simulink model "ADIA"  (R2018b)
settings: Solver=FixedStepDiscrete  StartTime=0.0  StopTime=10.0  FixedStep=0.02  RelTol=1e-3
undefined symbols (not defined in the file or in its folder): ACC_State_Active, ACC_State_BrakeOnly, ACC_State_Suspended, ACC_State_WaitingRise, ADAS_AEBBrakingProg, ADAS_DeclControlReq, ADAS_DriveOff, ADAS_ESCHoldReq_NotHold, ADASDecType_ACC, ADASDecType_AEB, ADIA_ACC_Acceleration_OOR_DecCount_C, ADIA_ACC_Acceleration_OOR_Duration_C, ADIA_ACC_Acceleration_OOR_IncCount_C, ADIA_ACC_Acceleration_OOR_LLim_C, ADIA_ACC_Acceleration_OOR_ULim_C, ADIA_ACC_AccelTrqReq_MixedDia_ULim_C, ADIA_ACC_AccelTrqReq_ULim_C, ADIA_ACC_Deceleration_Mixed_ULim_C, ADIA_ACC_Deceleration_OOR_DecCount_C, ADIA_ACC_Deceleration_OOR_Duration_C, ADIA_ACC_Deceleration_OOR_IncCount_C, ADIA_ACC_Deceleration_OOR_LLim_C, ADIA_ACC_Deceleration_OOR_ULim_C, ADIA_ACC_DriveOff_Distance_C, ADIA_ACC_DriveOff_TimeLim_C, ADIA_ACC_ReqMixed_DecCount_C, ADIA_ACC_ReqMixed_Duration_C, ADIA_ACC_ReqMixed_IncCount_C, ADIA_AccPedalRaw_MaxLim_C, ADIA_AccPedalRaw_MinLim_C, ADIA_ADAS_HoldDecReq_Set_C, ADIA_ADAS_HoldRConfirm_TimeLim_C, ADIA_ADAS_HoldVehSpd_Lim_C, ADIA_AEB_VehSpdDec_LLim_C, ADIA_AEB_VehSpdDec_ULim_C, ADIA_ASWFault_OvrdEn_C, ADIA_ASWFault_OvrdValue_C, ADIA_BatteryOutOfRange_DecCount_C, ADIA_BatteryOutOfRange_Duration_C, ADIA_BatteryOutOfRange_IncCount_C, ADIA_BattVolt_MaxLim_C, ADIA_BattVolt_MinLim_C, ADIA_BCM3_33C_InvBrkLight_DecCount_C, ADIA_BCM3_33C_InvBrkLight_Duration_C, ADIA_BCM3_33C_InvBrkLight_IncCount_C, ADIA_BCM_BattVolt_OvrdEn_C, ADIA_BCM_BattVolt_OvrdVal_C, ADIA_BCM_BrakeLampStaus_OvrdEn_C, ADIA_BCM_BrakeLampStaus_OvrdVal_C, ADIA_BCM_CHMSLStaus_OvrdEn_C, ADIA_BCM_CHMSLStaus_OvrdVal_C, ADIA_BCM_LeftTurnSwSt_OvrdEn_C, ADIA_BCM_LeftTurnSwSt_OvrdVal_C, ADIA_BCM_RightTurnSwSt_OvrdEn_C, ADIA_BCM_RightTurnSwSt_OvrdVal_C, ADIA_BCM_TurnSwFailure_DecCount_C, ADIA_BCM_TurnSwFailure_Duration_C, ADIA_BCM_TurnSwFailure_IncCount_C, ADIA_BSWFault_Ignore_C, ADIA_BSWFault_OvrdEn_C ... (+281)
libraries: simulink x208
(part 5 of 10)

== system ADIA/ADAS_Diagnostics/Diagnostics_Processing/DTC_ACC_HoldConfirm_Safety_Violation/Timer1 ==
  incrcondition : Inport
  incrvalue : Inport  Port=2
  decr condition : Inport  Port=3
  decvalue : Inport  Port=4
  maxlimit : Inport  Port=5
  reset : Inport  Port=6
  Constant{,1..3} (4 alike) : Constant  Value=0  OutDataTypeStr=Inherit: Inherit via back propagation
  MinMax1 : MinMax  Inputs=2  OutDataTypeStr=Inherit: Inherit via back propagation  InputSameDT=on
  MinMax2 : MinMax  Function=max  Inputs=2  OutDataTypeStr=Inherit: Inherit via back propagation  InputSameDT=on
  Relational Operator : RelationalOperator  OutDataTypeStr=boolean  RndMeth=Nearest
  Sum : Sum  Inputs=++-  OutDataTypeStr=Inherit: Inherit via back propagation  InputSameDT=on
  Unit Delay : UnitDelay  SampleTime=-1
  dec switch : Switch  Criteria=u2 ~= 0  Threshold=1  OutDataTypeStr=Inherit: Inherit via back propagation  InputSameDT=on
  inc switch : Switch  Criteria=u2 ~= 0  Threshold=1  OutDataTypeStr=Inherit: Inherit via back propagation  InputSameDT=on
  reset switch : Switch  Criteria=u2 ~= 0  Threshold=1  OutDataTypeStr=Inherit: Inherit via back propagation  InputSameDT=on
  counter out : Outport
  counter_status : Outport  Port=2
  wires:
  incrcondition/1 -> inc switch/2
  decr condition/1 -> dec switch/2
  Constant1/1 -> dec switch/3
  dec switch/1 -> Sum/3
  MinMax1/1 -> reset switch/3
  incrvalue/1 -> inc switch/1
  MinMax2/1 -> MinMax1/1
  Constant/1 -> inc switch/3
  reset/1 -> reset switch/2
  Unit Delay/1 -> Sum/1
  reset switch/1 -> Unit Delay/1, Relational Operator/1, counter out/1
  Constant2/1 -> MinMax2/1
  maxlimit/1 -> Relational Operator/2, MinMax1/2
  Sum/1 -> MinMax2/2
  inc switch/1 -> Sum/2
  Constant3/1 -> reset switch/1
  Relational Operator/1 -> counter_status/1
  decvalue/1 -> dec switch/1

== system ADIA/ADAS_Diagnostics/Diagnostics_Processing/DTC_ACC_Mixed_Mode_Conflict/Subsystem ==
  ADIAve_y_ADAS_DecelerationType : Inport  OutDataTypeStr=UInt8  PortDimensions=1
  ADIAve_g_ADAS_ACCTorqueReq : Inport  Port=2  OutDataTypeStr=T_M_Nm_Float32  PortDimensions=1
  ADIAve_g_ADAS_DecelerationSet : Inport  Port=3  OutDataTypeStr=T_M_Nm_Float32  PortDimensions=1
  Enable : EnablePort
  Constant1 : Constant  Value=ADIA_ACC_AccelTrqReq_MixedDia_ULim_C
  Constant10 : Constant  Value=SYS_False
  Constant11 : Constant  Value=Constant_0
  Constant4 : Constant  Value=ADIA_ACC_ReqMixed_DecCount_C
  Constant5 : Constant  Value=ADIA_ACC_ReqMixed_IncCount_C
  Constant6 : Constant  Value=ADIA_ACC_ReqMixed_Duration_C
  Constant8 : Constant  Value=ADASDecType_ACC
  Constant9 : Constant  Value=ADIA_ACC_Deceleration_Mixed_ULim_C
  "Latch " : Subsystem
  Logical Operator : Logic  AllPortsSameDT=off  OutDataTypeStr=boolean
  Logical Operator2 : Logic  Operator=NOT  AllPortsSameDT=off  OutDataTypeStr=boolean
  Logical Operator6 : Logic  AllPortsSameDT=off  OutDataTypeStr=boolean
  Relational Operator1 : RelationalOperator  Operator=>  OutDataTypeStr=boolean  RndMeth=Simplest
  Relational Operator4 : RelationalOperator  Operator===  OutDataTypeStr=boolean  RndMeth=Simplest
  Relational Operator6 : RelationalOperator  Operator===  OutDataTypeStr=boolean  RndMeth=Simplest
  Relational Operator7 : RelationalOperator  Operator=<  OutDataTypeStr=boolean  RndMeth=Simplest
  Timer1 : Subsystem
  ADIA_DTC_ACC_Mixed_Mode_Conflic : Outport
  wires:
  Logical Operator/1 -> Timer1/1(incrcondition), Logical Operator2/1
  Relational Operator6/1 -> Logical Operator6/1
  Logical Operator2/1 -> Timer1/3(decr condition)
  ADIAve_y_ADAS_DecelerationType/1 -> Relational Operator6/1
  "Latch "/1(Output) -> ADIA_DTC_ACC_Mixed_Mode_Conflic/1
  Constant5/1 -> Timer1/2(incrvalue)
  Relational Operator7/1 -> Logical Operator6/2
  Constant4/1 -> Timer1/4(decvalue)
  Constant11/1 -> Relational Operator4/2
  Constant9/1 -> Relational Operator7/2
  Constant6/1 -> Timer1/5(maxlimit)
  Timer1/1(counter out) -> Relational Operator4/1
  Constant10/1 -> Timer1/6(reset)
  Relational Operator4/1 -> "Latch "/2(Latch Reset)
  Timer1/2(counter_status) -> "Latch "/1(Input)
  Constant1/1 -> Relational Operator1/2
  ADIAve_g_ADAS_ACCTorqueReq/1 -> Relational Operator1/1
  Logical Operator6/1 -> Logical Operator/2
  Constant8/1 -> Relational Operator6/2
  ADIAve_g_ADAS_DecelerationSet/1 -> Relational Operator7/1
  Relational Operator1/1 -> Logical Operator/1

== system ADIA/ADAS_Diagnostics/Diagnostics_Processing/DTC_AEB_Safety_Violation/Latch 1 ==
  Input : Inport
  Latch Reset : Inport  Port=2
  Constant11 : Constant  Value=0  OutDataTypeStr=Inherit: Inherit via back propagation
  Constant12 : Constant  OutDataTypeStr=Inherit: Inherit via back propagation
  Switch : Switch  Threshold=1  OutDataTypeStr=Inherit: Inherit via back propagation  SaturateOnIntegerOverflow=on  InputSameDT=on
  Switch1 : Switch  Threshold=1  OutDataTypeStr=Inherit: Inherit via back propagation  SaturateOnIntegerOverflow=on  InputSameDT=on
  Unit Delay1 : UnitDelay  SampleTime=-1
  Output : Outport  InitialOutput=0
  wires:
  Constant12/1 -> Switch1/1
  Constant11/1 -> Switch/1
  Input/1 -> Switch1/2
  Unit Delay1/1 -> Switch1/3
  Switch/1 -> Unit Delay1/1, Output/1
  Latch Reset/1 -> Switch/2
  Switch1/1 -> Switch/3

== system ADIA/ADAS_Diagnostics/Diagnostics_Processing/DTC_AEB_Safety_Violation/Subsystem ==
  ADIAve_g_ESC_VeSpd : Inport  OutDataTypeStr=single  PortDimensions=1
  Enable : EnablePort
  ADIA_AEB_Begin_VehSpd : Outport
  wires:
  ADIAve_g_ESC_VeSpd/1 -> ADIA_AEB_Begin_VehSpd/1

== system ADIA/ADAS_Diagnostics/Diagnostics_Processing/DTC_AEB_Safety_Violation/Subsystem1 ==
  ADIAve_g_ESC_VeSpd : Inport  OutDataTypeStr=single  PortDimensions=1
  Enable : EnablePort
  ADIA_AEB_End_VehSpd : Outport
  wires:
  ADIAve_g_ESC_VeSpd/1 -> ADIA_AEB_End_VehSpd/1

== system ADIA/ADAS_Diagnostics/Diagnostics_Processing/Rationality_Diagnostics/ATFault ==
  Compare To Constant7 : simulink/Logic and Bit Operations/Compare To Constant  relop=~=  const=0  OutDataTypeStr=boolean
  Data Store Read51 : DataStoreRead  DataStoreName=ADIAve_y_TCU_ATFailure
  Event_FaultATFail : Outport
  wires:
  Compare To Constant7/1 -> Event_FaultATFail/1  "Event_FaulATFail4"
  Data Store Read51/1 -> Compare To Constant7/1  "ob_ADIAve_y_TCU_ATFailure"

== system ADIA/ADAS_Diagnostics/Diagnostics_Processing/Rationality_Diagnostics/BatteryOutOfRange ==
  Constant17 : Constant  Value=ADIA_BattVolt_MinLim_C
  Constant18 : Constant  Value=Constant_0
  Constant19 : Constant  Value=ADIA_BatteryOutOfRange_DecCount_C
  Constant20 : Constant  Value=ADIA_BatteryOutOfRange_IncCount_C
  Constant21 : Constant  Value=ADIA_BatteryOutOfRange_Duration_C
  Constant22 : Constant  Value=SYS_False
  Constant36 : Constant  Value=ADIA_BattVolt_MaxLim_C
  Counter&Latch : Subsystem
  Data Store Read34 : DataStoreRead  DataStoreName=ADIAve_g_BCM_BattVolt
  Logical Operator19 : Logic  Operator=OR  AllPortsSameDT=off  OutDataTypeStr=boolean
  Logical Operator20 : Logic  Operator=NOT  AllPortsSameDT=off  OutDataTypeStr=boolean
  Relational Operator15 : RelationalOperator  Operator=<  OutDataTypeStr=boolean  RndMeth=Simplest
  Relational Operator36 : RelationalOperator  Operator=>  OutDataTypeStr=boolean  RndMeth=Simplest
  "ADIA_DTC_BatteryOutOfRange " : Outport
  wires:
  Constant17/1 -> Relational Operator15/2
  Constant36/1 -> Relational Operator36/2
  Relational Operator36/1 -> Logical Operator19/2
  Relational Operator15/1 -> Logical Operator19/1
  Data Store Read34/1 -> Relational Operator36/1, Relational Operator15/1
  Logical Operator20/1 -> Counter&Latch/3(decrcondition)
  Logical Operator19/1 -> Counter&Latch/1(incrcondition), Logical Operator20/1
  Constant19/1 -> Counter&Latch/4(decvalue)
  Constant20/1 -> Counter&Latch/2(incrvalue)
  Constant18/1 -> Counter&Latch/7(LatchResetCounterVal)
  Constant21/1 -> Counter&Latch/5(maxlimit)
  Constant22/1 -> Counter&Latch/6(reset)
  Counter&Latch/1(Out1) -> "ADIA_DTC_BatteryOutOfRange "/1

== system ADIA/ADAS_Diagnostics/Diagnostics_Processing/Rationality_Diagnostics/CameraSystemError ==
  Constant18 : Constant  Value=Constant_0
  Constant19 : Constant  Value=ADIA_CameraSystemError_DecCount_C
  Constant20 : Constant  Value=ADIA_CameraSystemError_IncCount_C
  Constant21 : Constant  Value=ADIA_CameraSystemError_Duration_C
  Constant22 : Constant  Value=SYS_False
  Constant38 : Constant  Value=Camera_Status_OK
  Constant39 : Constant  Value=Camera_Status_Blocked
  Constant40 : Constant  Value=Camera_Status_Degraded
  Counter&Latch : Subsystem
  Data Store Read75 : DataStoreRead  DataStoreName=ADIAve_y_Camera_State
  Logical Operator1 : Logic  Inputs=3  AllPortsSameDT=off  OutDataTypeStr=boolean
  Logical Operator20 : Logic  Operator=NOT  AllPortsSameDT=off  OutDataTypeStr=boolean
  Relational Operator38 : RelationalOperator  Operator=~=  OutDataTypeStr=boolean  RndMeth=Simplest
  Relational Operator39 : RelationalOperator  Operator=~=  OutDataTypeStr=boolean  RndMeth=Simplest
  Relational Operator40 : RelationalOperator  Operator=~=  OutDataTypeStr=boolean  RndMeth=Simplest
  ADIA_DTC_CameraSystemError : Outport
  wires:
  Relational Operator39/1 -> Logical Operator1/2
  Constant39/1 -> Relational Operator39/2
  Constant40/1 -> Relational Operator40/2
  Relational Operator38/1 -> Logical Operator1/1
  Constant38/1 -> Relational Operator38/2
  Relational Operator40/1 -> Logical Operator1/3
  Data Store Read75/1 -> Relational Operator40/1, Relational Operator39/1, Relational Operator38/1  "ob_ADIAve_y_OperatingStatus"
  Logical Operator20/1 -> Counter&Latch/3(decrcondition)
  Logical Operator1/1 -> Logical Operator20/1, Counter&Latch/1(incrcondition)
  Constant19/1 -> Counter&Latch/4(decvalue)
  Constant20/1 -> Counter&Latch/2(incrvalue)
  Constant18/1 -> Counter&Latch/7(LatchResetCounterVal)
  Constant21/1 -> Counter&Latch/5(maxlimit)
  Constant22/1 -> Counter&Latch/6(reset)
  Counter&Latch/1(Out1) -> ADIA_DTC_CameraSystemError/1

== system ADIA/ADAS_Diagnostics/Diagnostics_Processing/Rationality_Diagnostics/DTC_BCM3_33C_InvBrkLight ==
  Constant18 : Constant  Value=Constant_0
  Constant19 : Constant  Value=ADIA_BCM3_33C_InvBrkLight_DecCount_C
  Constant20 : Constant  Value=ADIA_BCM3_33C_InvBrkLight_IncCount_C
  Constant21 : Constant  Value=ADIA_BCM3_33C_InvBrkLight_Duration_C
  Constant22 : Constant  Value=SYS_False
  Constant24 : Constant  Value=BCM_BrakeLamp_Invalid
  Constant3 : Constant  Value=BCM_BrakeLamp_Fault
  Counter&Latch : Subsystem
  Data Store Read55 : DataStoreRead  DataStoreName=ADIAve_y_BCM_CHMSLStaus
  Data Store Read56 : DataStoreRead  DataStoreName=ADIAve_y_BCM_BrakeLampStaus
  Logical Operator2 : Logic  Operator=OR  AllPortsSameDT=off  OutDataTypeStr=boolean
  Logical Operator20 : Logic  Operator=NOT  AllPortsSameDT=off  OutDataTypeStr=boolean
  Logical Operator3 : Logic  Operator=OR  AllPortsSameDT=off  OutDataTypeStr=boolean
  Logical Operator8 : Logic  Operator=OR  AllPortsSameDT=off  OutDataTypeStr=boolean
  Relational Operator{21..24} (4 alike) : RelationalOperator  Operator===  OutDataTypeStr=boolean  RndMeth=Simplest
  ADIA_DTC_BCM3_33C_InvBrkLight : Outport
  wires:
  Relational Operator22/1 -> Logical Operator2/2
  Constant3/1 -> Relational Operator21/2, Relational Operator23/2
  Relational Operator23/1 -> Logical Operator3/1
  Logical Operator2/1 -> Logical Operator8/1
  Logical Operator3/1 -> Logical Operator8/2
  Relational Operator21/1 -> Logical Operator2/1
  Constant24/1 -> Relational Operator22/2, Relational Operator24/2
  Data Store Read56/1 -> Relational Operator23/1, Relational Operator24/1
  Data Store Read55/1 -> Relational Operator22/1, Relational Operator21/1
  Relational Operator24/1 -> Logical Operator3/2
  Logical Operator20/1 -> Counter&Latch/3(decrcondition)
  Logical Operator8/1 -> Counter&Latch/1(incrcondition), Logical Operator20/1
  Constant19/1 -> Counter&Latch/4(decvalue)
  Constant20/1 -> Counter&Latch/2(incrvalue)
  Constant18/1 -> Counter&Latch/7(LatchResetCounterVal)
  Constant21/1 -> Counter&Latch/5(maxlimit)
  Constant22/1 -> Counter&Latch/6(reset)
  Counter&Latch/1(Out1) -> ADIA_DTC_BCM3_33C_InvBrkLight/1

== system ADIA/ADAS_Diagnostics/Diagnostics_Processing/Rationality_Diagnostics/DTC_EMS_14A_OorACCStatus ==
  Constant18 : Constant  Value=Constant_0
  Constant19 : Constant  Value=ADIA_EMS_14A_OorACCStatus_DecCount_C
  Constant20 : Constant  Value=ADIA_EMS_14A_OorACCStatus_IncCount_C
  Constant21 : Constant  Value=ADIA_EMS_14A_OorACCStatus_Duration_C
  Constant22 : Constant  Value=SYS_False
  Constant25 : Constant  Value=EMS_ACCResponse_Reserved
  Constant26 : Constant  Value=ADIA_EMS_ACCResponse_MaxLim_C
  Counter&Latch : Subsystem
  Data Store Read54 : DataStoreRead  DataStoreName=ADIAve_y_EMS_ACCResponseStatus
  Logical Operator20 : Logic  Operator=NOT  AllPortsSameDT=off  OutDataTypeStr=boolean
  Logical Operator5 : Logic  Operator=OR  AllPortsSameDT=off  OutDataTypeStr=boolean
  Relational Operator25 : RelationalOperator  Operator===  OutDataTypeStr=boolean  RndMeth=Simplest
  Relational Operator26 : RelationalOperator  Operator=>  OutDataTypeStr=boolean  RndMeth=Simplest
  ADIA_DTC_EMS_14A_OorACCStatus : Outport
  wires:
  Data Store Read54/1 -> Relational Operator26/1, Relational Operator25/1  "ob_ADIAve_y_EMS_ACCResponseStatus"
  Constant25/1 -> Relational Operator25/2
  Relational Operator26/1 -> Logical Operator5/1
  Constant26/1 -> Relational Operator26/2
  Relational Operator25/1 -> Logical Operator5/2
  Logical Operator20/1 -> Counter&Latch/3(decrcondition)
  Logical Operator5/1 -> Counter&Latch/1(incrcondition), Logical Operator20/1
  Constant19/1 -> Counter&Latch/4(decvalue)
  Constant20/1 -> Counter&Latch/2(incrvalue)
  Constant18/1 -> Counter&Latch/7(LatchResetCounterVal)
  Constant21/1 -> Counter&Latch/5(maxlimit)
  Constant22/1 -> Counter&Latch/6(reset)
  Counter&Latch/1(Out1) -> ADIA_DTC_EMS_14A_OorACCStatus/1

== system ADIA/ADAS_Diagnostics/Diagnostics_Processing/Rationality_Diagnostics/DTC_WheelSpdFaultSignal ==
  Compare To Constant{1..4} (4 alike) : simulink/Logic and Bit Operations/Compare To Constant  relop=~=  const=0  OutDataTypeStr=boolean
  Constant18 : Constant  Value=Constant_0
  Constant19 : Constant  Value=ADIA_WhlSpdFaultSignal_DecCount_C
  Constant20 : Constant  Value=ADIA_WhlSpdFaultSignal_IncCount_C
  Constant21 : Constant  Value=ADIA_WhlSpdFaultSignal_Duration_C
  Constant22 : Constant  Value=SYS_False
  Counter&Latch : Subsystem
  Data Store Read46 : DataStoreRead  DataStoreName=ADIAve_y_ESC_FLWhlSpdFaultSignal
  Data Store Read47 : DataStoreRead  DataStoreName=ADIAve_y_ESC_FRWhlSpdFaultSignal
  Data Store Read48 : DataStoreRead  DataStoreName=ADIAve_y_ESC_RLWhlSpdFaultSignal
  Data Store Read49 : DataStoreRead  DataStoreName=ADIAve_y_ESC_RRWhlSpdFaultSignal
  Logical Operator : Logic  Operator=OR  Inputs=4  AllPortsSameDT=off  OutDataTypeStr=boolean
  Logical Operator20 : Logic  Operator=NOT  AllPortsSameDT=off  OutDataTypeStr=boolean
  ADIA_DTC_WheelSpdFaultSignal : Outport
  wires:
  Compare To Constant1/1 -> Logical Operator/1
  Logical Operator/1 -> Logical Operator20/1, Counter&Latch/1(incrcondition)
  Constant22/1 -> Counter&Latch/6(reset)
  Constant21/1 -> Counter&Latch/5(maxlimit)
  Data Store Read47/1 -> Compare To Constant2/1  "ob_ADIAve_y_ESC_FRWHeelSpdFaultSignal"
  Compare To Constant2/1 -> Logical Operator/2
  Compare To Constant3/1 -> Logical Operator/3
  Constant18/1 -> Counter&Latch/7(LatchResetCounterVal)
  Constant19/1 -> Counter&Latch/4(decvalue)
  Constant20/1 -> Counter&Latch/2(incrvalue)
  Counter&Latch/1(Out1) -> ADIA_DTC_WheelSpdFaultSignal/1
  Logical Operator20/1 -> Counter&Latch/3(decrcondition)
  Data Store Read46/1 -> Compare To Constant1/1  "ob_ADIAve_y_ESC_FLWHeelSpdFaultSignal"
  Data Store Read49/1 -> Compare To Constant4/1  "ob_ADIAve_y_ESC_RRWHeelSpdFaultSignal"
  Data Store Read48/1 -> Compare To Constant3/1  "ob_ADIAve_y_ESC_RLWHeelSpdFaultSignal"
  Compare To Constant4/1 -> Logical Operator/4

== system ADIA/ADAS_Diagnostics/Diagnostics_Processing/Rationality_Diagnostics/EMS10_88_InvAccPedPosRaw ==
  Constant13 : Constant  Value=ADIA_AccPedalRaw_MaxLim_C
  Constant18 : Constant  Value=Constant_0
  Constant19 : Constant  Value=ADIA_EMS10_88_InvAccPedPosRaw_DecCount_C
  Constant20 : Constant  Value=ADIA_EMS10_88_InvAccPedPosRaw_IncCount_C
  Constant21 : Constant  Value=ADIA_EMS10_88_InvAccPedPosRaw_Duration_C
  Constant22 : Constant  Value=SYS_False
  Constant27 : Constant  Value=ADIA_AccPedalRaw_MinLim_C
  Counter&Latch : Subsystem
  Data Store Read42 : DataStoreRead  DataStoreName=ADIAve_g_EMS_AccPdPositionRaw
  Logical Operator18 : Logic  Operator=OR  AllPortsSameDT=off  OutDataTypeStr=boolean
  Logical Operator20 : Logic  Operator=NOT  AllPortsSameDT=off  OutDataTypeStr=boolean
  Relational Operator11 : RelationalOperator  Operator=>  OutDataTypeStr=boolean  RndMeth=Simplest
  Relational Operator27 : RelationalOperator  Operator=<  OutDataTypeStr=boolean  RndMeth=Simplest
  ADIA_DTC_EMS10_88_InvAccPedPosRaw : Outport
  wires:
  Constant27/1 -> Relational Operator27/2
  Data Store Read42/1 -> Relational Operator27/1, Relational Operator11/1
  Relational Operator27/1 -> Logical Operator18/2
  Relational Operator11/1 -> Logical Operator18/1
  Constant13/1 -> Relational Operator11/2
  Logical Operator20/1 -> Counter&Latch/3(decrcondition)
  Logical Operator18/1 -> Counter&Latch/1(incrcondition), Logical Operator20/1
  Constant19/1 -> Counter&Latch/4(decvalue)
  Constant20/1 -> Counter&Latch/2(incrvalue)
  Constant18/1 -> Counter&Latch/7(LatchResetCounterVal)
  Constant21/1 -> Counter&Latch/5(maxlimit)
  Constant22/1 -> Counter&Latch/6(reset)
  Counter&Latch/1(Out1) -> ADIA_DTC_EMS10_88_InvAccPedPosRaw/1

== system ADIA/ADAS_Diagnostics/Diagnostics_Processing/Rationality_Diagnostics/EMS5_E0_InvOorBrkPedal ==
  Constant18 : Constant  Value=Constant_0
  Constant19 : Constant  Value=ADIA_EMS5_E0_InvOorBrkPedal_DecCount_C
  Constant20 : Constant  Value=ADIA_EMS5_E0_InvOorBrkPedal_IncCount_C
  Constant21 : Constant  Value=ADIA_EMS5_E0_InvOorBrkPedal_Duration_C
  Constant22 : Constant  Value=SYS_False
  Constant28 : Constant  Value=EMS_BrakePedal_Fault
  Counter&Latch : Subsystem
  Data Store Read72 : DataStoreRead  DataStoreName=ADIAve_y_EMS_BrakePedalSignal
  Logical Operator20 : Logic  Operator=NOT  AllPortsSameDT=off  OutDataTypeStr=boolean
  Relational Operator28 : RelationalOperator  Operator===  OutDataTypeStr=boolean  RndMeth=Simplest
  ADIA_DTC_EMS5_E0_InvOorBrkPedal : Outport
  wires:
  Constant28/1 -> Relational Operator28/2
  Data Store Read72/1 -> Relational Operator28/1  "ob_ADIAve_y_EMS_BrakePedalSignal"
  Logical Operator20/1 -> Counter&Latch/3(decrcondition)
  Relational Operator28/1 -> Counter&Latch/1(incrcondition), Logical Operator20/1
  Constant19/1 -> Counter&Latch/4(decvalue)
  Constant20/1 -> Counter&Latch/2(incrvalue)
  Constant18/1 -> Counter&Latch/7(LatchResetCounterVal)
  Constant21/1 -> Counter&Latch/5(maxlimit)
  Constant22/1 -> Counter&Latch/6(reset)
  Counter&Latch/1(Out1) -> ADIA_DTC_EMS5_E0_InvOorBrkPedal/1

== system ADIA/ADAS_Diagnostics/Diagnostics_Processing/Rationality_Diagnostics/EMS5_E0_OorEngineStas ==
  Constant18 : Constant  Value=Constant_0
  Constant19 : Constant  Value=ADIA_EMS5_E0_OorEngineStas_DecCount_C
  Constant20 : Constant  Value=ADIA_EMS5_E0_OorEngineStas_IncCount_C
  Constant21 : Constant  Value=ADIA_EMS5_E0_OorEngineStas_Duration_C
  Constant22 : Constant  Value=SYS_False
  Constant29 : Constant  Value=EMS_EngStatus_MaxLim
  Counter&Latch : Subsystem
  Data Store Read57 : DataStoreRead  DataStoreName=ADIAve_y_EMS_EngRunningStatus
  Logical Operator20 : Logic  Operator=NOT  AllPortsSameDT=off  OutDataTypeStr=boolean
  Relational Operator29 : RelationalOperator  Operator=>  OutDataTypeStr=boolean  RndMeth=Simplest
  ADIA_DTC_EMS5_E0_OorEngineStas : Outport
  wires:
  Constant29/1 -> Relational Operator29/2
  Data Store Read57/1 -> Relational Operator29/1  "ob_ADIAve_y_EMS_EngRunningStatus"
  Logical Operator20/1 -> Counter&Latch/3(decrcondition)
  Relational Operator29/1 -> Logical Operator20/1, Counter&Latch/1(incrcondition)
  Constant19/1 -> Counter&Latch/4(decvalue)
  Constant20/1 -> Counter&Latch/2(incrvalue)
  Constant18/1 -> Counter&Latch/7(LatchResetCounterVal)
  Constant21/1 -> Counter&Latch/5(maxlimit)
  Constant22/1 -> Counter&Latch/6(reset)
  Counter&Latch/1(Out1) -> ADIA_DTC_EMS5_E0_OorEngineStas/1

== system ADIA/ADAS_Diagnostics/Diagnostics_Processing/Rationality_Diagnostics/EMS_14B_InvOorRealWhlTrq ==
  Constant : Constant  Value=ADIA_EMS_RealWhlTrq_MinLim_C
  Constant18 : Constant  Value=Constant_0
  Constant19 : Constant  Value=ADIA_EMS_14B_InvOorRealWhlTrq_DecCount_C
  Constant2 : Constant  Value=ADIA_EMS_RealWhlTrq_MaxLim_C
  Constant20 : Constant  Value=ADIA_EMS_14B_InvOorRealWhlTrq_IncCount_C
  Constant21 : Constant  Value=ADIA_EMS_14B_InvOorRealWhlTrq_Duration_C
  Constant22 : Constant  Value=SYS_False
  Counter&Latch : Subsystem
  Data Store Read79 : DataStoreRead  DataStoreName=ADIAve_d_EMS_RealPTWhlTrq
  Logical Operator20 : Logic  Operator=NOT  AllPortsSameDT=off  OutDataTypeStr=boolean
  Logical Operator9 : Logic  Operator=OR  AllPortsSameDT=off  OutDataTypeStr=boolean
  Relational Operator : RelationalOperator  Operator=<  OutDataTypeStr=boolean  RndMeth=Simplest
  Relational Operator1 : RelationalOperator  Operator=>  OutDataTypeStr=boolean  RndMeth=Simplest
  ADIA_DTC_EMS_14B_InvOorRealWhlTrq : Outport
  wires:
  Constant2/1 -> Relational Operator1/2
  Relational Operator/1 -> Logical Operator9/2
  Data Store Read79/1 -> Relational Operator1/1, Relational Operator/1
  Relational Operator1/1 -> Logical Operator9/1
  Constant/1 -> Relational Operator/2
  Logical Operator20/1 -> Counter&Latch/3(decrcondition)
  Logical Operator9/1 -> Logical Operator20/1, Counter&Latch/1(incrcondition)
  Constant19/1 -> Counter&Latch/4(decvalue)
  Constant20/1 -> Counter&Latch/2(incrvalue)
  Constant18/1 -> Counter&Latch/7(LatchResetCounterVal)
  Constant21/1 -> Counter&Latch/5(maxlimit)
  Constant22/1 -> Counter&Latch/6(reset)
  Counter&Latch/1(Out1) -> ADIA_DTC_EMS_14B_InvOorRealWhlTrq/1

== system ADIA/ADAS_Diagnostics/Diagnostics_Processing/Rationality_Diagnostics/EMS_17E_InvOorMaxNoCtrlTrq ==
  Constant18 : Constant  Value=Constant_0
  Constant19 : Constant  Value=ADIA_EMS_17E_InvOorMaxNoCtrlTrq_DecCount_C
  Constant20 : Constant  Value=ADIA_EMS_17E_InvOorMaxNoCtrlTrq_IncCount_C
  Constant21 : Constant  Value=ADIA_EMS_17E_InvOorMaxNoCtrlTrq_Duration_C
  Constant22 : Constant  Value=SYS_False
  Constant5 : Constant  Value=ADIA_EMS_MaxNoCtrlWhlTrqOst_MinLim_C
  Constant6 : Constant  Value=ADIA_EMS_MaxNoCtrlWhlTrqOst_MaxLim_C
  Counter&Latch : Subsystem
  Data Store Read80 : DataStoreRead  DataStoreName=ADIAve_g_EMS_MaxNoCtrlWhlTrqOst
  Logical Operator10 : Logic  Operator=OR  AllPortsSameDT=off  OutDataTypeStr=boolean
  Logical Operator20 : Logic  Operator=NOT  AllPortsSameDT=off  OutDataTypeStr=boolean
  Relational Operator2 : RelationalOperator  Operator=<  OutDataTypeStr=boolean  RndMeth=Simplest
  Relational Operator3 : RelationalOperator  Operator=>  OutDataTypeStr=boolean  RndMeth=Simplest
  ADIA_DTC_EMS_17E_InvOorMaxNoCtrlTrq : Outport
  wires:
  Relational Operator2/1 -> Logical Operator10/2
  Constant5/1 -> Relational Operator2/2
  Relational Operator3/1 -> Logical Operator10/1
  Data Store Read80/1 -> Relational Operator2/1, Relational Operator3/1
  Constant6/1 -> Relational Operator3/2
  Logical Operator20/1 -> Counter&Latch/3(decrcondition)
  Logical Operator10/1 -> Counter&Latch/1(incrcondition), Logical Operator20/1
  Constant19/1 -> Counter&Latch/4(decvalue)
  Constant20/1 -> Counter&Latch/2(incrvalue)
  Constant18/1 -> Counter&Latch/7(LatchResetCounterVal)
  Constant21/1 -> Counter&Latch/5(maxlimit)
  Constant22/1 -> Counter&Latch/6(reset)
  Counter&Latch/1(Out1) -> ADIA_DTC_EMS_17E_InvOorMaxNoCtrlTrq/1

== system ADIA/ADAS_Diagnostics/Diagnostics_Processing/Rationality_Diagnostics/EMS_17E_InvOorMaxTrqWhl ==
  Constant18 : Constant  Value=Constant_0
  Constant19 : Constant  Value=ADIA_EMS_17E_InvOorMaxTrqWhl_DecCount_C
  Constant20 : Constant  Value=ADIA_EMS_17E_InvOorMaxTrqWhl_IncCount_C
  Constant21 : Constant  Value=ADIA_EMS_17E_InvOorMaxTrqWhl_Duration_C
  Constant22 : Constant  Value=SYS_False
  Constant7 : Constant  Value=ADIA_EMS_MaxWhlTrq_MaxLim_C
  Constant8 : Constant  Value=ADIA_EMS_MaxWhlTrq_MinLim_C
  Counter&Latch : Subsystem
  Data Store Read81 : DataStoreRead  DataStoreName=ADIAve_g_EMS_MaxWhlTrq
  Logical Operator11 : Logic  Operator=OR  AllPortsSameDT=off  OutDataTypeStr=boolean
  Logical Operator20 : Logic  Operator=NOT  AllPortsSameDT=off  OutDataTypeStr=boolean
  Relational Operator4 : RelationalOperator  Operator=<  OutDataTypeStr=boolean  RndMeth=Simplest
  Relational Operator5 : RelationalOperator  Operator=>  OutDataTypeStr=boolean  RndMeth=Simplest
  ADIA_DTC_EMS_17E_InvOorMaxTrqWhl : Outport
  wires:
  Constant7/1 -> Relational Operator5/2
  Relational Operator5/1 -> Logical Operator11/1
  Data Store Read81/1 -> Relational Operator4/1, Relational Operator5/1
  Relational Operator4/1 -> Logical Operator11/2
  Constant8/1 -> Relational Operator4/2
  Logical Operator20/1 -> Counter&Latch/3(decrcondition)
  Logical Operator11/1 -> Logical Operator20/1, Counter&Latch/1(incrcondition)
  Constant19/1 -> Counter&Latch/4(decvalue)
  Constant20/1 -> Counter&Latch/2(incrvalue)
  Constant18/1 -> Counter&Latch/7(LatchResetCounterVal)
  Constant21/1 -> Counter&Latch/5(maxlimit)
  Constant22/1 -> Counter&Latch/6(reset)
  Counter&Latch/1(Out1) -> ADIA_DTC_EMS_17E_InvOorMaxTrqWhl/1

== system ADIA/ADAS_Diagnostics/Diagnostics_Processing/Rationality_Diagnostics/EMS_17E_InvOorMinNoCtrlTrq ==
  Constant10 : Constant  Value=ADIA_EMS_MinNoCtrlWhlTrqOst_MaxLim_C
  Constant18 : Constant  Value=Constant_0
  Constant19 : Constant  Value=ADIA_EMS_17E_InvOorMinNoCtrlTrq_DecCount_C
  Constant20 : Constant  Value=ADIA_EMS_17E_InvOorMinNoCtrlTrq_IncCount_C
  Constant21 : Constant  Value=ADIA_EMS_17E_InvOorMinNoCtrlTrq_Duration_C
  Constant22 : Constant  Value=SYS_False
  Constant9 : Constant  Value=ADIA_EMS_MinNoCtrlWhlTrqOst_MinLim_C
  Counter&Latch : Subsystem
  Data Store Read44 : DataStoreRead  DataStoreName=ADIAve_g_EMS_MinNoCtrlWhlTrqOst
  Logical Operator12 : Logic  Operator=OR  AllPortsSameDT=off  OutDataTypeStr=boolean
  Logical Operator20 : Logic  Operator=NOT  AllPortsSameDT=off  OutDataTypeStr=boolean
  Relational Operator6 : RelationalOperator  Operator=<  OutDataTypeStr=boolean  RndMeth=Simplest
  Relational Operator7 : RelationalOperator  Operator=>  OutDataTypeStr=boolean  RndMeth=Simplest
  ADIA_DTC_EMS_17E_InvOorMinNotContrlWhlTrq : Outport
  wires:
  Data Store Read44/1 -> Relational Operator6/1, Relational Operator7/1
  Relational Operator7/1 -> Logical Operator12/1
  Constant9/1 -> Relational Operator6/2
  Relational Operator6/1 -> Logical Operator12/2
  Constant10/1 -> Relational Operator7/2
  Logical Operator20/1 -> Counter&Latch/3(decrcondition)
  Logical Operator12/1 -> Logical Operator20/1, Counter&Latch/1(incrcondition)
  Constant19/1 -> Counter&Latch/4(decvalue)
  Constant20/1 -> Counter&Latch/2(incrvalue)
  Constant18/1 -> Counter&Latch/7(LatchResetCounterVal)
  Constant21/1 -> Counter&Latch/5(maxlimit)
  Constant22/1 -> Counter&Latch/6(reset)
  Counter&Latch/1(Out1) -> ADIA_DTC_EMS_17E_InvOorMinNotContrlWhlTrq/1

== system ADIA/ADAS_Diagnostics/Diagnostics_Processing/Rationality_Diagnostics/EMS_17E_InvOorMinTrqWhl ==
  Constant11 : Constant  Value=ADIA_EMS_MinWhlTrq_MaxLim_C
  Constant12 : Constant  Value=ADIA_EMS_MinWhlTrq_MinLim_C
  Constant18 : Constant  Value=Constant_0
  Constant19 : Constant  Value=ADIA_EMS_17E_InvOorMinTrqWhl_DecCount_C
  Constant20 : Constant  Value=ADIA_EMS_17E_InvOorMinTrqWhl_IncCount_C
  Constant21 : Constant  Value=ADIA_EMS_17E_InvOorMinTrqWhl_Duration_C
  Constant22 : Constant  Value=SYS_False
  Counter&Latch : Subsystem
  Data Store Read43 : DataStoreRead  DataStoreName=ADIAve_g_EMS_MinWhlTrq
  Logical Operator13 : Logic  Operator=OR  AllPortsSameDT=off  OutDataTypeStr=boolean
  Logical Operator20 : Logic  Operator=NOT  AllPortsSameDT=off  OutDataTypeStr=boolean
  Relational Operator8 : RelationalOperator  Operator=<  OutDataTypeStr=boolean  RndMeth=Simplest
  Relational Operator9 : RelationalOperator  Operator=>  OutDataTypeStr=boolean  RndMeth=Simplest
  ADIA_DTC_EMS_17E_InvOorMinTrqWhl : Outport
  wires:
  Data Store Read43/1 -> Relational Operator8/1, Relational Operator9/1
  Constant11/1 -> Relational Operator9/2
  Constant12/1 -> Relational Operator8/2
  Relational Operator9/1 -> Logical Operator13/1
  Relational Operator8/1 -> Logical Operator13/2
  Logical Operator20/1 -> Counter&Latch/3(decrcondition)
  Logical Operator13/1 -> Logical Operator20/1, Counter&Latch/1(incrcondition)
  Constant19/1 -> Counter&Latch/4(decvalue)
  Constant20/1 -> Counter&Latch/2(incrvalue)
  Constant18/1 -> Counter&Latch/7(LatchResetCounterVal)
  Constant21/1 -> Counter&Latch/5(maxlimit)
  Constant22/1 -> Counter&Latch/6(reset)
  Counter&Latch/1(Out1) -> ADIA_DTC_EMS_17E_InvOorMinTrqWhl/1

== system ADIA/ADAS_Diagnostics/Diagnostics_Processing/Rationality_Diagnostics/EPS2_17A_InvOorSteAngle ==
  note: 0：Invalid1：Valid
  Abs : Abs
  Compare To Constant34 : simulink/Logic and Bit Operations/Compare To Constant  relop===  const=0  OutDataTypeStr=boolean
  Constant18 : Constant  Value=Constant_0
  Constant19 : Constant  Value=ADIA_EPS2_17A_InvOorSteAngle_DecCount_C
  Constant20 : Constant  Value=ADIA_EPS2_17A_InvOorSteAngle_IncCount_C
  Constant21 : Constant  Value=ADIA_EPS2_17A_InvOorSteAngle_Duration_C
  Constant22 : Constant  Value=SYS_False
  Constant30 : Constant  Value=ADIA_EPS_SteerAngle_MaxLim_C
  Counter&Latch : Subsystem
  Data Store Read30 : DataStoreRead  DataStoreName=ADIAve_g_EPS_SteerAngle
  Data Store Read60 : DataStoreRead  DataStoreName=ADIAve_y_EPS_SteeringAngle_Flag
  Logical Operator14 : Logic  Operator=OR  AllPortsSameDT=off  OutDataTypeStr=boolean
  Logical Operator20 : Logic  Operator=NOT  AllPortsSameDT=off  OutDataTypeStr=boolean
  Relational Operator30 : RelationalOperator  Operator=>  OutDataTypeStr=boolean  RndMeth=Simplest
  ADIA_DTC_EPS2_17A_InvOorSteAngle : Outport
  wires:
  Abs/1 -> Relational Operator30/1
  Constant30/1 -> Relational Operator30/2
  Data Store Read30/1 -> Abs/1
  Data Store Read60/1 -> Compare To Constant34/1
  Relational Operator30/1 -> Logical Operator14/2
  Compare To Constant34/1 -> Logical Operator14/1
  Logical Operator20/1 -> Counter&Latch/3(decrcondition)
  Logical Operator14/1 -> Logical Operator20/1, Counter&Latch/1(incrcondition)
  Constant19/1 -> Counter&Latch/4(decvalue)
  Constant20/1 -> Counter&Latch/2(incrvalue)
  Constant18/1 -> Counter&Latch/7(LatchResetCounterVal)
  Constant21/1 -> Counter&Latch/5(maxlimit)
  Constant22/1 -> Counter&Latch/6(reset)
  Counter&Latch/1(Out1) -> ADIA_DTC_EPS2_17A_InvOorSteAngle/1

== system ADIA/ADAS_Diagnostics/Diagnostics_Processing/Rationality_Diagnostics/EPS2_17A_InvStTorq ==
  note: 0：正常1：异常
  Abs1 : Abs
  Compare To Constant5 : simulink/Logic and Bit Operations/Compare To Constant  relop=~=  const=0  OutDataTypeStr=boolean
  Constant18 : Constant  Value=Constant_0
  Constant19 : Constant  Value=ADIA_EPS2_17A_InvStTorq_DecCount_C
  Constant20 : Constant  Value=ADIA_EPS2_17A_InvStTorq_IncCount_C
  Constant21 : Constant  Value=ADIA_EPS2_17A_InvStTorq_Duration_C
  Constant22 : Constant  Value=SYS_False
  Constant31 : Constant  Value=ADIA_EPS_SteerTorque_MaxLim_C
  Counter&Latch : Subsystem
  Data Store Read41 : DataStoreRead  DataStoreName=ADIAve_g_EPS_SteerTrq
  Data Store Read50 : DataStoreRead  DataStoreName=ADIAve_y_EPS_SteerTrqSensorSt
  Logical Operator15 : Logic  Operator=OR  AllPortsSameDT=off  OutDataTypeStr=boolean
  Logical Operator20 : Logic  Operator=NOT  AllPortsSameDT=off  OutDataTypeStr=boolean
  Relational Operator31 : RelationalOperator  Operator=>  OutDataTypeStr=boolean  RndMeth=Simplest
  ADIA_DTC_EPS2_17A_InvStTorq : Outport
  wires:
  Data Store Read41/1 -> Abs1/1
  Abs1/1 -> Relational Operator31/1
  Constant31/1 -> Relational Operator31/2
  Relational Operator31/1 -> Logical Operator15/2
  Compare To Constant5/1 -> Logical Operator15/1
  Data Store Read50/1 -> Compare To Constant5/1  "ob_ADIAve_y_EPS_SteerintTorqueSensorSt"
  Logical Operator20/1 -> Counter&Latch/3(decrcondition)
  Logical Operator15/1 -> Counter&Latch/1(incrcondition), Logical Operator20/1
  Constant19/1 -> Counter&Latch/4(decvalue)
  Constant20/1 -> Counter&Latch/2(incrvalue)
  Constant18/1 -> Counter&Latch/7(LatchResetCounterVal)
  Constant21/1 -> Counter&Latch/5(maxlimit)
  Constant22/1 -> Counter&Latch/6(reset)
  Counter&Latch/1(Out1) -> ADIA_DTC_EPS2_17A_InvStTorq/1

== system ADIA/ADAS_Diagnostics/Diagnostics_Processing/Rationality_Diagnostics/EPS3_31C_InvOorLKAState ==
  Constant18 : Constant  Value=Constant_0
  Constant19 : Constant  Value=ADIA_EPS3_31C_InvOorLKAState_DecCount_C
  Constant20 : Constant  Value=ADIA_EPS3_31C_InvOorLKAState_IncCount_C
  Constant21 : Constant  Value=ADIA_EPS3_31C_InvOorLKAState_Duration_C
  Constant22 : Constant  Value=SYS_False
  Constant32 : Constant  Value=EPS_LKAState_Defect
  Counter&Latch : Subsystem
  Data Store Read59 : DataStoreRead  DataStoreName=ADIAve_y_EPS_LKAState
  Logical Operator20 : Logic  Operator=NOT  AllPortsSameDT=off  OutDataTypeStr=boolean
  Relational Operator32 : RelationalOperator  Operator===  OutDataTypeStr=boolean  RndMeth=Simplest
  ADIA_DTC_EPS3_31C_InvOorLKAState : Outport
  wires:
  Data Store Read59/1 -> Relational Operator32/1  "ob_ADIAve_y_EPS_LKAState"
  Constant32/1 -> Relational Operator32/2
  Logical Operator20/1 -> Counter&Latch/3(decrcondition)
  Relational Operator32/1 -> Counter&Latch/1(incrcondition), Logical Operator20/1
  Constant19/1 -> Counter&Latch/4(decvalue)
  Constant20/1 -> Counter&Latch/2(incrvalue)
  Constant18/1 -> Counter&Latch/7(LatchResetCounterVal)
  Constant21/1 -> Counter&Latch/5(maxlimit)
  Constant22/1 -> Counter&Latch/6(reset)
  Counter&Latch/1(Out1) -> ADIA_DTC_EPS3_31C_InvOorLKAState/1

== system ADIA/ADAS_Diagnostics/Diagnostics_Processing/Rationality_Diagnostics/ESC2_A0_InvOorVehSpeed ==
  note: 0:无错误（ No Fault）1: 错误（Fault）
  Compare To Constant35 : simulink/Logic and Bit Operations/Compare To Constant  relop=~=  const=0  OutDataTypeStr=boolean
  Constant18 : Constant  Value=Constant_0
  Constant19 : Constant  Value=ADIA_ESC2_A0_InvOorVehSpeed_DecCount_C
  Constant20 : Constant  Value=ADIA_ESC2_A0_InvOorVehSpeed_IncCount_C
  Constant21 : Constant  Value=ADIA_ESC2_A0_InvOorVehSpeed_Duration_C
  Constant22 : Constant  Value=SYS_False
  Constant33 : Constant  Value=ADIA_ESC_VehSpd_MaxLim_C
  Counter&Latch : Subsystem
  Data Store Read26 : DataStoreRead  DataStoreName=ADIAve_g_ESC_VehSpd
  Data Store Read45 : DataStoreRead  DataStoreName=ADIAve_y_ESC_VehSpdValidFlag
  Logical Operator16 : Logic  Operator=OR  AllPortsSameDT=off  OutDataTypeStr=boolean
  Logical Operator20 : Logic  Operator=NOT  AllPortsSameDT=off  OutDataTypeStr=boolean
  Relational Operator33 : RelationalOperator  Operator=>  OutDataTypeStr=boolean  RndMeth=Simplest
  ADIA_DTC_ESC2_A0_InvOorVehSpeed : Outport
  wires:
  Data Store Read26/1 -> Relational Operator33/1
  Data Store Read45/1 -> Compare To Constant35/1  "ob_ADIAve_y_ESC_VehSpdValidFlag"
  Compare To Constant35/1 -> Logical Operator16/1
  Relational Operator33/1 -> Logical Operator16/2
  Constant33/1 -> Relational Operator33/2
  Logical Operator20/1 -> Counter&Latch/3(decrcondition)
  Logical Operator16/1 -> Counter&Latch/1(incrcondition), Logical Operator20/1
  Constant19/1 -> Counter&Latch/4(decvalue)
  Constant20/1 -> Counter&Latch/2(incrvalue)
  Constant18/1 -> Counter&Latch/7(LatchResetCounterVal)
  Constant21/1 -> Counter&Latch/5(maxlimit)
  Constant22/1 -> Counter&Latch/6(reset)
  Counter&Latch/1(Out1) -> ADIA_DTC_ESC2_A0_InvOorVehSpeed/1

== system ADIA/ADAS_Diagnostics/Diagnostics_Processing/Rationality_Diagnostics/ESC3_121_InvOorTCSActive ==
  note: 0：工作1：不工作2：错误
  Compare To Constant23 : simulink/Logic and Bit Operations/Compare To Constant  relop===  const=2  OutDataTypeStr=boolean
  Constant18 : Constant  Value=Constant_0
  Constant19 : Constant  Value=ADIA_ESC3_121_InvOorTCSActive_DecCount_C
  Constant20 : Constant  Value=ADIA_ESC3_121_InvOorTCSActive_IncCount_C
  Constant21 : Constant  Value=ADIA_ESC3_121_InvOorTCSActive_Duration_C
  Constant22 : Constant  Value=SYS_False
  Counter&Latch : Subsystem
  Data Store Read61 : DataStoreRead  DataStoreName=ADIAve_y_ESC_TCSCtlActive
  Logical Operator20 : Logic  Operator=NOT  AllPortsSameDT=off  OutDataTypeStr=boolean
  ADIA_DTC_ESC3_121_InvOorTCSActive : Outport
  wires:
  Compare To Constant23/1 -> Logical Operator20/1, Counter&Latch/1(incrcondition)  "Event_OutRangeHoldSta_SetEventStatus22"
  Data Store Read61/1 -> Compare To Constant23/1  "ob_ADIAve_y_ESC_TCSCtlActive"
  Logical Operator20/1 -> Counter&Latch/3(decrcondition)
  Constant19/1 -> Counter&Latch/4(decvalue)
  Constant20/1 -> Counter&Latch/2(incrvalue)
  Constant18/1 -> Counter&Latch/7(LatchResetCounterVal)
  Constant21/1 -> Counter&Latch/5(maxlimit)
  Constant22/1 -> Counter&Latch/6(reset)
  Counter&Latch/1(Out1) -> ADIA_DTC_ESC3_121_InvOorTCSActive/1

== system ADIA/ADAS_Diagnostics/Diagnostics_Processing/Rationality_Diagnostics/ESC3_121_InvOorVehStand ==
  note: 0：standstill1：not standstill2：invalid
  Compare To Constant10 : simulink/Logic and Bit Operations/Compare To Constant  relop===  const=2  OutDataTypeStr=boolean
  Constant18 : Constant  Value=Constant_0
  Constant19 : Constant  Value=ADIA_ESC3_121_InvOorVehStand_DecCount_C
  Constant20 : Constant  Value=ADIA_ESC3_121_InvOorVehStand_IncCount_C
  Constant21 : Constant  Value=ADIA_ESC3_121_InvOorVehStand_Duration_C
  Constant22 : Constant  Value=SYS_False
  Counter&Latch : Subsystem
  Data Store Read63 : DataStoreRead  DataStoreName=ADIAve_y_ESC_VehicleStandstill
  Logical Operator20 : Logic  Operator=NOT  AllPortsSameDT=off  OutDataTypeStr=boolean
  ADIA_DTC_ESC3_121_InvOorVehStandstill : Outport
  wires:
  Data Store Read63/1 -> Compare To Constant10/1  "ob_ADIAve_y_ESC_VehicleStandstill"
  Compare To Constant10/1 -> Counter&Latch/1(incrcondition), Logical Operator20/1  "Event_OutRangePowStrSta_SetEventStatus19"
  Logical Operator20/1 -> Counter&Latch/3(decrcondition)
  Constant19/1 -> Counter&Latch/4(decvalue)
  Constant20/1 -> Counter&Latch/2(incrvalue)
  Constant18/1 -> Counter&Latch/7(LatchResetCounterVal)
  Constant21/1 -> Counter&Latch/5(maxlimit)
  Constant22/1 -> Counter&Latch/6(reset)
  Counter&Latch/1(Out1) -> ADIA_DTC_ESC3_121_InvOorVehStandstill/1

== system ADIA/ADAS_Diagnostics/Diagnostics_Processing/Rationality_Diagnostics/ESC5_122_InvOorLatAccel ==
  note: 0：有效1：无效
  Compare To Constant19 : simulink/Logic and Bit Operations/Compare To Constant  relop===  const=1  OutDataTypeStr=boolean
  Constant18 : Constant  Value=Constant_0
  Constant19 : Constant  Value=ADIA_ESC5_122_InvOorLatAccel_DecCount_C
  Constant20 : Constant  Value=ADIA_ESC5_122_InvOorLatAccel_IncCount_C
  Constant21 : Constant  Value=ADIA_ESC5_122_InvOorLatAccel_Duration_C
  Constant22 : Constant  Value=SYS_False
  Counter&Latch : Subsystem
  Data Store Read65 : DataStoreRead  DataStoreName=ADIAve_y_ESC_LateralAccelValidity
  Logical Operator20 : Logic  Operator=NOT  AllPortsSameDT=off  OutDataTypeStr=boolean
  ADIA_DTC_ESC5_122_InvOorLatAccel : Outport
  wires:
  Compare To Constant19/1 -> Logical Operator20/1, Counter&Latch/1(incrcondition)  "Event_OutRangePowStrSta_SetEventStatus19"
  Data Store Read65/1 -> Compare To Constant19/1  "ob_ADIAve_y_ESC_LateralAccelarationValidity"
  Logical Operator20/1 -> Counter&Latch/3(decrcondition)
  Constant19/1 -> Counter&Latch/4(decvalue)
  Constant20/1 -> Counter&Latch/2(incrvalue)
  Constant18/1 -> Counter&Latch/7(LatchResetCounterVal)
  Constant21/1 -> Counter&Latch/5(maxlimit)
  Constant22/1 -> Counter&Latch/6(reset)
  Counter&Latch/1(Out1) -> ADIA_DTC_ESC5_122_InvOorLatAccel/1

== system ADIA/ADAS_Diagnostics/Diagnostics_Processing/Rationality_Diagnostics/ESC5_122_InvOorLongiAccel ==
  Compare To Constant21 : simulink/Logic and Bit Operations/Compare To Constant  relop===  const=1  OutDataTypeStr=boolean
  Constant18 : Constant  Value=Constant_0
  Constant19 : Constant  Value=ADIA_ESC5_122_InvOorLongiAccel_DecCount_C
  Constant20 : Constant  Value=ADIA_ESC5_122_InvOorLongiAccel_IncCount_C
  Constant21 : Constant  Value=ADIA_ESC5_122_InvOorLongiAccel_Duration_C
  Constant22 : Constant  Value=SYS_False
  Counter&Latch : Subsystem
  Data Store Read66 : DataStoreRead  DataStoreName=ADIAve_y_ESC_LongitudinalAccelValidity
  Logical Operator20 : Logic  Operator=NOT  AllPortsSameDT=off  OutDataTypeStr=boolean
  ADIA_DTC_ESC5_122_InvOorLongiAccel : Outport
  wires:
  Compare To Constant21/1 -> Logical Operator20/1, Counter&Latch/1(incrcondition)  "Event_OutRangePowStrSta_SetEventStatus19"
  Data Store Read66/1 -> Compare To Constant21/1  "ob_ADIAve_y_ESC_LongitudinalAccelervalidity"
  Logical Operator20/1 -> Counter&Latch/3(decrcondition)
  Constant19/1 -> Counter&Latch/4(decvalue)
  Constant20/1 -> Counter&Latch/2(incrvalue)
  Constant18/1 -> Counter&Latch/7(LatchResetCounterVal)
  Constant21/1 -> Counter&Latch/5(maxlimit)
  Constant22/1 -> Counter&Latch/6(reset)
  Counter&Latch/1(Out1) -> ADIA_DTC_ESC5_122_InvOorLongiAccel/1

== system ADIA/ADAS_Diagnostics/Diagnostics_Processing/Rationality_Diagnostics/ESC5_122_InvOorStaticSlope ==
  Abs2 : Abs
  Constant18 : Constant  Value=Constant_0
  Constant19 : Constant  Value=ADIA_ESC5_122_InvOorStaticSlope_DecCount_C
  Constant20 : Constant  Value=ADIA_ESC5_122_InvOorStaticSlope_IncCount_C
  Constant21 : Constant  Value=ADIA_ESC5_122_InvOorStaticSlope_Duration_C
  Constant22 : Constant  Value=SYS_False
  Constant34 : Constant  Value=ADIA_ESC_StaticSlope_MaxLim_C
  Counter&Latch : Subsystem
  Data Store Read32 : DataStoreRead  DataStoreName=ADIAve_y_ESC_StaticSlope
  Logical Operator20 : Logic  Operator=NOT  AllPortsSameDT=off  OutDataTypeStr=boolean
  Relational Operator10 : RelationalOperator  Operator=>  OutDataTypeStr=boolean  RndMeth=Simplest
  ADIA_DTC_ESC5_122_InvOorStaticSlope : Outport
  wires:
  Constant34/1 -> Relational Operator10/2
  Data Store Read32/1 -> Abs2/1
  Abs2/1 -> Relational Operator10/1
  Logical Operator20/1 -> Counter&Latch/3(decrcondition)
  Relational Operator10/1 -> Logical Operator20/1, Counter&Latch/1(incrcondition)
  Constant19/1 -> Counter&Latch/4(decvalue)
  Constant20/1 -> Counter&Latch/2(incrvalue)
  Constant18/1 -> Counter&Latch/7(LatchResetCounterVal)
  Constant21/1 -> Counter&Latch/5(maxlimit)
  Constant22/1 -> Counter&Latch/6(reset)
  Counter&Latch/1(Out1) -> ADIA_DTC_ESC5_122_InvOorStaticSlope/1

== system ADIA/ADAS_Diagnostics/Diagnostics_Processing/Rationality_Diagnostics/ESC5_122_InvOorYawRate ==
  Abs3 : Abs
  Compare To Constant11 : simulink/Logic and Bit Operations/Compare To Constant  relop===  const=1  OutDataTypeStr=boolean
  Constant14 : Constant  Value=ADIA_ESC_YawRate_MaxLim_C
  Constant18 : Constant  Value=Constant_0
  Constant19 : Constant  Value=ADIA_ESC5_122_InvOorYawRate_DecCount_C
  Constant20 : Constant  Value=ADIA_ESC5_122_InvOorYawRate_IncCount_C
  Constant21 : Constant  Value=ADIA_ESC5_122_InvOorYawRate_Duration_C
  Constant22 : Constant  Value=SYS_False
  Counter&Latch : Subsystem
  Data Store Read29 : DataStoreRead  DataStoreName=ADIAve_g_ESC_YawRate
  Data Store Read64 : DataStoreRead  DataStoreName=ADIAve_y_ESC_YawrateValidity
  Logical Operator17 : Logic  Operator=OR  AllPortsSameDT=off  OutDataTypeStr=boolean
  Logical Operator20 : Logic  Operator=NOT  AllPortsSameDT=off  OutDataTypeStr=boolean
  Relational Operator34 : RelationalOperator  Operator=>  OutDataTypeStr=boolean  RndMeth=Simplest
  ADIA_DTC_ESC5_122_InvOorYawRate : Outport
  wires:
  Compare To Constant11/1 -> Logical Operator17/1  "Event_OutRangePowStrSta_SetEventStatus19"
  Abs3/1 -> Relational Operator34/1
  Data Store Read29/1 -> Abs3/1
  Relational Operator34/1 -> Logical Operator17/2
  Data Store Read64/1 -> Compare To Constant11/1  "ob_ADIAve_y_ESC_YawrateValidity"
  Constant14/1 -> Relational Operator34/2
  Logical Operator20/1 -> Counter&Latch/3(decrcondition)
  Logical Operator17/1 -> Counter&Latch/1(incrcondition), Logical Operator20/1
  Constant19/1 -> Counter&Latch/4(decvalue)
  Constant20/1 -> Counter&Latch/2(incrvalue)
  Constant18/1 -> Counter&Latch/7(LatchResetCounterVal)
  Constant21/1 -> Counter&Latch/5(maxlimit)
  Constant22/1 -> Counter&Latch/6(reset)
  Counter&Latch/1(Out1) -> ADIA_DTC_ESC5_122_InvOorYawRate/1

== system ADIA/ADAS_Diagnostics/Diagnostics_Processing/Rationality_Diagnostics/ESC6_123_InvOorDynSlope ==
  Abs5 : Abs
  Constant18 : Constant  Value=Constant_0
  Constant19 : Constant  Value=ADIA_ESC6_123_InvOorDynSlope_DecCount_C
  Constant20 : Constant  Value=ADIA_ESC6_123_InvOorDynSlope_IncCount_C
  Constant21 : Constant  Value=ADIA_ESC6_123_InvOorDynSlope_Duration_C
  Constant22 : Constant  Value=SYS_False
  Constant35 : Constant  Value=ADIA_ESC_DynSlope_MaxLim_C
  Counter&Latch : Subsystem
  Data Store Read31 : DataStoreRead  DataStoreName=ADIAve_y_ESC_DynSlope
  Logical Operator20 : Logic  Operator=NOT  AllPortsSameDT=off  OutDataTypeStr=boolean
  Relational Operator35 : RelationalOperator  Operator=>  OutDataTypeStr=boolean  RndMeth=Simplest
  ADIA_DTC_ESC6_123_InvOorDynSlope : Outport
  wires:
  Data Store Read31/1 -> Abs5/1
  Abs5/1 -> Relational Operator35/1
  Constant35/1 -> Relational Operator35/2
  Logical Operator20/1 -> Counter&Latch/3(decrcondition)
  Relational Operator35/1 -> Counter&Latch/1(incrcondition), Logical Operator20/1
  Constant19/1 -> Counter&Latch/4(decvalue)
  Constant20/1 -> Counter&Latch/2(incrvalue)
  Constant18/1 -> Counter&Latch/7(LatchResetCounterVal)
  Constant21/1 -> Counter&Latch/5(maxlimit)
  Constant22/1 -> Counter&Latch/6(reset)
  Counter&Latch/1(Out1) -> ADIA_DTC_ESC6_123_InvOorDynSlope/1

== system ADIA/ADAS_Diagnostics/Diagnostics_Processing/Rationality_Diagnostics/ESC6_123_InvUnfilYawRate ==
  Abs4 : Abs
  Constant18 : Constant  Value=Constant_0
  Constant19 : Constant  Value=ADIA_ESC6_123_InvUnfilYawRate_DecCount_C
  Constant20 : Constant  Value=ADIA_ESC6_123_InvUnfilYawRate_IncCount_C
  Constant21 : Constant  Value=ADIA_ESC6_123_InvUnfilYawRate_Duration_C
  Constant22 : Constant  Value=SYS_False
  Constant4 : Constant  Value=ADIA_ESC_UnfltYawRate_MaxLim_C
  Counter&Latch : Subsystem
  Data Store Read40 : DataStoreRead  DataStoreName=ADIAve_g_ESC_UnfltYawRate
  Logical Operator20 : Logic  Operator=NOT  AllPortsSameDT=off  OutDataTypeStr=boolean
  Relational Operator12 : RelationalOperator  Operator=>  OutDataTypeStr=boolean  RndMeth=Simplest
  ADIA_DTC_ESC6_123_InvUnfilYawRate : Outport
  wires:
  Constant4/1 -> Relational Operator12/2
  Data Store Read40/1 -> Abs4/1
  Abs4/1 -> Relational Operator12/1
  Logical Operator20/1 -> Counter&Latch/3(decrcondition)
  Relational Operator12/1 -> Logical Operator20/1, Counter&Latch/1(incrcondition)
  Constant19/1 -> Counter&Latch/4(decvalue)
  Constant20/1 -> Counter&Latch/2(incrvalue)
  Constant18/1 -> Counter&Latch/7(LatchResetCounterVal)
  Constant21/1 -> Counter&Latch/5(maxlimit)
  Constant22/1 -> Counter&Latch/6(reset)
  Counter&Latch/1(Out1) -> ADIA_DTC_ESC6_123_InvUnfilYawRate/1
